simulink model "PasseBas"  (R2021b)
settings: Solver=VariableStepAuto  StartTime=0.0  StopTime=10  RelTol=1e-3
undefined symbols (not defined in the file): fdesignblkfcn, gcbh
libraries: dspspect3 x1, dspvision x1, dspobslib x1
settings Model: Creator=coren  LastModifiedBy=coren

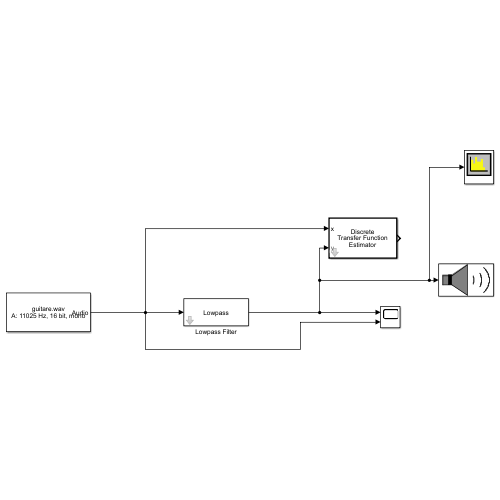
[thumbnail: Simulink's stored preview of the top-level diagram]
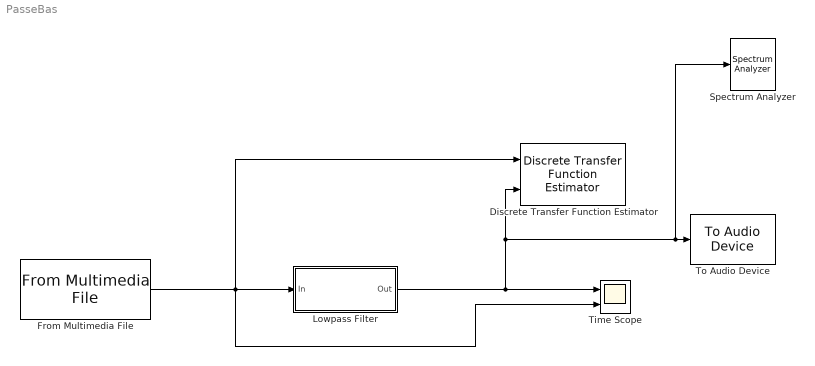
== system PasseBas ==
  Discrete Transfer Function Estimator : dspspect3/Discrete Transfer Function Estimator  WindowMode=Specify on dialog  WindowLength=1024  Overlap=50  AveragingMethod=Running  ForgettingFactorPort=off  ForgettingFactor=0.9  SpectralAverages=100  FFTLengthSource=Auto  FFTLength=128  Window=Hann  SidelobeAttenuation=60  FrequencyRange=One-sided  OutputCoherence=off  SimulateUsing=Code generation
      settings: SourceProductBaseCode=DS
  From Multimedia File : dspvision/From Multimedia File  inputFilename=C:\Users\coren\Documents\MATLAB\Traitement Images et Son 3E105\Projet Son\guitare.wav  readRange=[1 Inf]  loop=on  numPlays=inf  outputStreams=Audio only  videoDataType=single  audioDataType=double  inheritSampleTime=on  userDefinedSampleTime=1/30  noAudioOutput=off  isIntensityVideo=off  fourcc=RGB  colorVideoFormat=Separate color signals  outputEOF=off  dataOrg=Column-major  audioFrameSize=1024  computeAudioFrameSize=off  outSamplingMode=Sample based
  Lowpass Filter : Subsystem  DialogController=fdesignblkfcn  InitFcn=fdesignblkfcn(gcbh, {'InitFcn'});  mask(Lowpass Filter){}
      mask help: Design a lowpass filter
      settings: CopyFcn=fdesignblkfcn(gcbh, {'CopyFcn'});
      mask Help: helpview(mapfilelocation('dsp'), 'dsplowpassfilter');
      mask Display: disp('Lowpass')
  Spectrum Analyzer : SpectrumAnalyzer
  Time Scope : Scope  NumInputPorts=2
  To Audio Device : dspobslib/To Audio Device  deviceName=Default  inheritSampleRate=on  sampleRate=44100  deviceDatatype=Determine from input data type  autoBufferSize=on  bufferSize=4096  queueDuration=1.0  defaultOutputChannelMapping=on  outputChannelMapping=1:2  outputNumUnderrunSamples=off
      settings: SourceProductBaseCode=DS
  wires:
  Lowpass Filter/1(Out) -> Spectrum Analyzer/1, To Audio Device/1, Discrete Transfer Function Estimator/2, Time Scope/1
  From Multimedia File/1 -> Lowpass Filter/1(In), Time Scope/2, Discrete Transfer Function Estimator/1

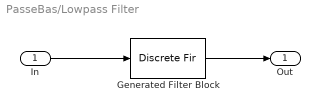
== system PasseBas/Lowpass Filter ==
  In : Inport
  Generated Filter Block : DiscreteFir  Tag=BlockMethodSubSystem  Coefficients=[-0.000412827868467195887 9.81243430181901979e-05 0.000832486305851584197 0.00133122445047580162 0.00064851716000773464 -0.00135196933841895926 -0.00325822334745372614 -0.00281654522597758143 0.000944497817461176638 0.00587645652010064523 0.00739720026398984435 0.00217378238033037394 -0.00777364730965379985 -0.0146673757842439474 -0.0102641722420114545 0.00615262607745049612 0.0238758733277565985 0.0262781191062598056 0.00403400806006494386 -0.033171105434620575 -0.0570640376350071768 -0.0365034199845649457 0.0401379236603261538 0.151610910309707886 0.250902401807135356 0.290605618620347728 0.250902401807135356 0.151610910309707886 0.0401379236603261538 -0.0365034199845649457 -0.0570640376350071768 -0.033171105434620575 0.00403400806006494386 0.0262781191062598056 0.0238758733277565985 0.00615262607745049612 -0.0102641722420114545 -0.0146673757842439474 -0.00777364730965379985 0.00217378238033037394 0.00739720026398984435 0.00587645652010064523 0.000944497817461176638 -0.00281654522597758143 -0.00325822334745372614 -0.00135196933841895926 0.00064851716000773464 0.00133122445047580162 0.000832486305851584197 9.81243430181901979e-05 -0.000412827868467195887]  InputProcessing=Columns as channels (frame based)
  Out : Outport
  wires:
  Generated Filter Block/1 -> Out/1
  In/1 -> Generated Filter Block/1
